simulink model "Underactuated_PFL_SMC"  (R2024b)
settings: Solver=FixedStepAuto  StartTime=0.0  StopTime=50  FixedStep=0.0001  RelTol=1e-3
settings Model: Creator=olive  LastModifiedBy=olivermcnaughton
settings DebuggingCC: UnderSpecifiedDimensionMsg=warning

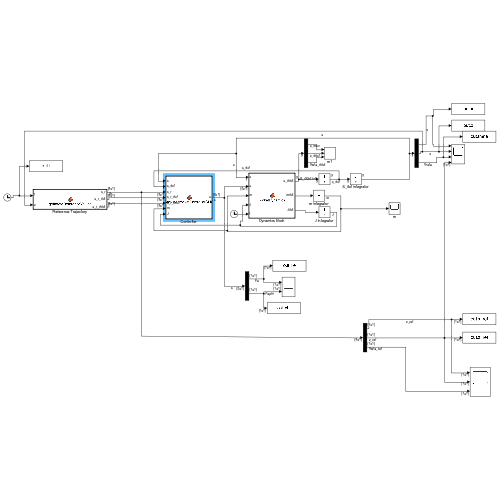
[thumbnail: Simulink's stored preview of the top-level diagram]
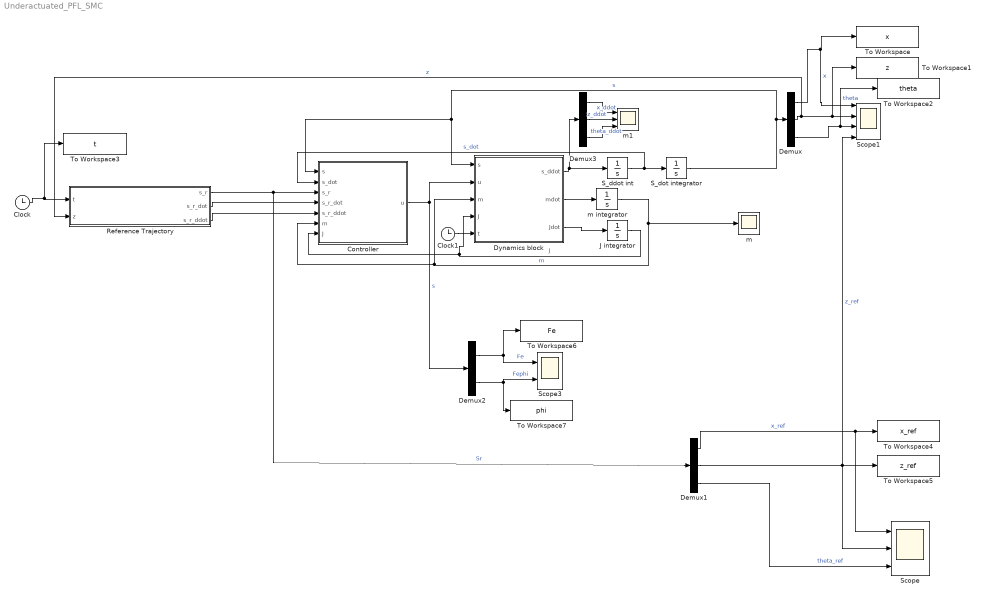
== system Underactuated_PFL_SMC ==
  Clock : Clock
  Clock1 : Clock
  Controller : MATLAB Function  TreatAsAtomicUnit=on
  Demux : Demux  Outputs=3
  Demux1 : Demux  Outputs=3
  Demux2 : Demux  Outputs=2
  Demux3 : Demux  Outputs=3
  Dynamics block : MATLAB Function  TreatAsAtomicUnit=on
  J integrator : Integrator  InitialCondition=5
  Reference Trajectory : MATLAB Function  TreatAsAtomicUnit=on
  S_ddot int : Integrator  InitialCondition=[0; 0; 0]
  S_dot integrator : Integrator  InitialCondition=[0;0;0]
  Scope : Scope  NumInputPorts=3
  Scope1 : Scope  NumInputPorts=4
  Scope3 : Scope  NumInputPorts=2
  To Workspace : ToWorkspace  VariableName=x  SaveFormat=Timeseries  SampleTime=-1
  To Workspace1 : ToWorkspace  VariableName=z  SaveFormat=Timeseries  SampleTime=-1
  To Workspace2 : ToWorkspace  VariableName=theta  SaveFormat=Timeseries  SampleTime=-1
  To Workspace3 : ToWorkspace  VariableName=t  SaveFormat=Timeseries  SampleTime=-1
  To Workspace4 : ToWorkspace  VariableName=x_ref  SaveFormat=Timeseries  SampleTime=-1
  To Workspace5 : ToWorkspace  VariableName=z_ref  SaveFormat=Timeseries  SampleTime=-1
  To Workspace6 : ToWorkspace  VariableName=Fe  SaveFormat=Timeseries  SampleTime=-1
  To Workspace7 : ToWorkspace  VariableName=phi  SaveFormat=Timeseries  SampleTime=-1
  m : Scope
  m integrator : Integrator  InitialCondition=25
  m1 : Scope  NumInputPorts=3
  wires:
  Dynamics block/1(s_ddot) -> Demux3/1, S_ddot int/1
  Dynamics block/2(mdot) -> m integrator/1
  Dynamics block/3(Jdot) -> J integrator/1
  S_ddot int/1 -> Controller/2(s_dot), S_dot integrator/1  "s_dot"
  S_dot integrator/1 -> Controller/1(s), Dynamics block/1(s), Demux/1  "s"
  J integrator/1 -> Dynamics block/4(J), Controller/7(J)  "J"
  m integrator/1 -> Dynamics block/3(m), Controller/6(m), m/1  "m"
  Demux/1 -> To Workspace/1, Scope1/1  "x"
  Demux/2 -> Reference Trajectory/2(z), To Workspace1/1, Scope1/2  "z"
  Demux/3 -> To Workspace2/1, Scope1/3  "theta"
  Demux2/2 -> To Workspace7/1, Scope3/2  "Fephi"
  Demux2/1 -> To Workspace6/1, Scope3/1  "Fe"
  Controller/1(u) -> Dynamics block/2(u), Demux2/1  "s"
  Clock/1 -> To Workspace3/1, Reference Trajectory/1(t)
  Reference Trajectory/1(s_r) -> Demux1/1, Controller/3(s_r)  "Sr"
  Demux1/2 -> To Workspace5/1, Scope1/4, Scope/2  "z_ref"
  Demux1/1 -> Scope/1, To Workspace4/1  "x_ref"
  Demux1/3 -> Scope/3  "theta_ref"
  Reference Trajectory/2(s_r_dot) -> Controller/4(s_r_dot)
  Demux3/1 -> m1/1  "x_ddot"
  Demux3/2 -> m1/2  "z_ddot"
  Demux3/3 -> m1/3  "theta_ddot"
  Reference Trajectory/3(s_r_ddot) -> Controller/5(s_r_ddot)
  Clock1/1 -> Dynamics block/5(t)

== matlab function Underactuated_PFL_SMC/Reference Trajectory ==
  data: s_r output; s_r_dot output; t input; z input; s_r_ddot output
function [s_r, s_r_dot, s_r_ddot] = generateReferenceValues(t,z)
% Generates constant reference position and velocity values for x, z, and theta
% Outputs:
%   sr: Reference position vector [x_ref; z_ref; theta_ref]
%   srdot: Reference velocity vector [x_dot_ref; z_dot_ref; theta_dot_ref]

%set position and time for each segment
%set to 1 for a hover, set 0 otherwise
hover = 1;
%set to 1 if tuning
if hover ==1
    x_ref = 2;
    z_ref = 2;
    theta_ref = 0;

    x_dot_ref = 0;
    z_dot_ref = 0;
    theta_dot_ref = 0;

    x_ddot_ref = 0;
    z_ddot_ref = 0;
    theta_ddot_ref = 0;
else
    %the rocket follows a trajectory of a half sine wave (middle part) then a
    %semi circle for the top of the boostback portion 
    %then a straight line downwards
    %End time of half sinewave
    T1 = 10;
    %End point of half sine wave
    x1 = 30;
    z1 = 40;
    
    %End time of semi circle 
    T2 = 20;
    %End point of semi circle
    x2 = 15; %gives you the position of the other side of the semi circle
    z2 = 40; %this should equal z1
    
    %Landing time of rocket
    T3 = 50;
    
    % Initialize reference values for safety
    x_ref = 0;
    z_ref = 0;
    theta_ref = 0;

    x_dot_ref = 0;
    z_dot_ref = 0;
    theta_dot_ref = 0;

    x_ddot_ref = 0;
    z_ddot_ref = 0;
    theta_ddot_ref = 0;

    %The first half sine wave
    if t<T1
        %reference positions
        x_ref = (-sin((pi/2) + pi*t/T1)+1)*x1/2;
        z_ref = z1*t/T1;
        theta_ref = atan(sin(pi*t/T1));
        
        %Reference Velocities
        x_dot_ref = (-pi/T1)*cos((pi/2) + pi*t/T1)*x1/2;
        z_dot_ref = z1/T1;
        theta_dot_ref = (pi/T1)*cos(pi*t/T1)/(sin(pi*t/T1)^2 + 1);

        %Reference Accelerations
        x_ddot_ref = ((pi/T1)^2)*sin((pi/2) + pi*t/T1)*x1/2;
        z_ddot_ref = 0;
        k = pi/T1;
        theta_ddot_ref = -k^2 * sin(k * t) * (3 - sin(k * t)^2) / (1 + sin(k * t)^2)^2;
    end
    %now doing the semi circle
    if t<T2 && t>=T1
        %calculate radius
        r = (x1-x2)/2; %radius 
        h = (x1+x2)/2; %x position for centre of circle
        dT = T2-T1; %Time between points
        dX = x1-x2;
        thetaMax = pi/4; %max angle at when halfway through the semi circle 
        teff = t -T1; %need to "zero" compared to the RHS of the semi circle
        %reference positions
        x_ref = h + r*cos(pi*teff/dT);
        z_ref = z1 + r*sin(pi*teff/dT);
        theta_ref = thetaMax*sin(2*pi*teff/dT + pi);
        %Reference Velocities
        x_dot_ref = (-pi/dT)*r*sin(pi*teff/dT);
        z_dot_ref = (pi/dT)*r*cos(pi*teff/dT);
        theta_dot_ref = thetaMax*(2*pi/dT)*cos(2*pi*teff/dT + pi);

        %Reference Accelerations
        x_ddot_ref = -(pi^2/dT^2)*r*cos(pi*teff/dT);
        z_ddot_ref = -(pi^2/dT^2)*r*sin(pi*teff/dT);
        theta_ddot_ref = -4*(pi^2/dT^2)*thetaMax*sin(pi*teff/dT + pi);
    end
    %now it is landing
    if t>=T2 
        % Position
        x_ref = x2; % Assuming no horizontal movement during landing
        z_ref = z2-4*(t-T2);
        theta_ref = 0; % No rotation during landing
        
        % Velocity
        x_dot_ref = 0;
        if z<10
            z_dot_ref = 0;
            z_ref = 5;
        else 
            z_dot_ref = -4;
        end
        
        theta_dot_ref = 0;
        
        % Acceleration
        x_ddot_ref = 0;
        z_ddot_ref = 0;
        theta_ddot_ref = 0;
    end
    if t>T3
        x_ref = x2;
        z_ref = 5;
        theta_ref = 0; % No rotation during landing
    end
    
end
% Output reference values
s_r = [x_ref; z_ref; theta_ref];
s_r_dot = [x_dot_ref; z_dot_ref; theta_dot_ref];
s_r_ddot = [x_ddot_ref; z_ddot_ref; theta_ddot_ref];
end

== matlab function Underactuated_PFL_SMC/Dynamics block ==
  data: s input size=3; u input; m input; J input; s_ddot output size=3; mdot output size=1; Jdot output size=1; t input
function [s_ddot,mdot,Jdot] = rocketDynamics(s,u,m,J,t)

%initialise states
L1 = 1;
alpha1 = 0.009;
alpha2 = 0.005;
beta = 0.03;
g = 9.81;

%extract states
Fe = u(1);
phi = u(2);
theta = s(3);

%find mdot and Jdot
mdot = -alpha1*(beta*Fe);
Jdot = -alpha2*(beta*Fe);

% Disturbances 
Fx_dist = 20*sin(0.5*t);    %N     
Fz_dist = 20*sin(0.5*t);    %N
M_dist  = 20*sin(0.5*t);    %(Nm)

% Maybe the actual mass is 20% heavier than the "m" we pass to the controller
m_actual = 1 * m; 

%acclerations 
x_ddot     = (Fe*sin(theta + phi) + Fx_dist) / m_actual;
z_ddot     = -g + (Fe*cos(theta + phi) + Fz_dist) / m_actual;
theta_ddot = (Fe*sin(phi)*L1 + M_dist) / J;

s_ddot = [x_ddot;z_ddot;theta_ddot];

end

== matlab function Underactuated_PFL_SMC/Controller ==
  data: s input; s_dot input; s_r input; s_r_dot input; s_r_ddot input; m input; J input; u output
function u = BacksteprocketControllerSMC(s, s_dot, s_r, s_r_dot, s_r_ddot, m, J)
% rocketController - Backstepping-based + Sliding Mode Control for rocket dynamics

% Define bounds
FE_min = 0;   % Lower bound for FE
FE_max = 500; % Upper bound for FE
phi_min = -pi/6;  % Lower bound for phi
phi_max = pi/6;   % Upper bound for phi

% Constants
g = 9.81; % Gravity

% Extract current states
x = s(1);
z = s(2);
theta = s(3);
x_dot = s_dot(1);
z_dot = s_dot(2);
theta_dot = s_dot(3);

% Extract reference states
x_ref = s_r(1);
z_ref = s_r(2);
theta_ref = s_r(3);
x_dot_ref = s_r_dot(1);
z_dot_ref = s_r_dot(2);
theta_dot_ref = s_r_dot(3);
x_ddot_ref = s_r_ddot(1);
z_ddot_ref = s_r_ddot(2);
theta_ddot_ref = s_r_ddot(3);

% Control gains (Backstepping)
%proportional | Derivative
kpx = 2;        kdx = 5;
kpz = 2;        kdz = 5;
kpt = 1;        kdt = 1;

% Sliding Mode Gains
lambda_x = 0.1;  % Tuning parameter for x sliding surface
lambda_z = 0.1;  % Tuning parameter for z sliding surface
lambda_t = 0.1;  % Tuning parameter for theta sliding surface

eta_x = 10;    % SMC gain for x
eta_z = 0.1;    % SMC gain for z
eta_t = 0.1;     % SMC gain for theta

psi_x = 1;
psi_z = 1;
psi_t = 1;

% Define Sliding Surfaces
ex = x - x_ref;
ez = z - z_ref;
et = theta - theta_ref;
edotx = x_dot - x_dot_ref;
edotz = z_dot - z_dot_ref;
edot_t = theta_dot - theta_dot_ref;

sx = edotx + lambda_x * ex;  % Sliding surface for x
sz = edotz + lambda_z * ez;  % Sliding surface for z
st = edot_t + lambda_t * et; % Sliding surface for theta

% Smooth Sliding Mode Control (Using Tanh Function)
SMC_x = -eta_x * tanh(sx / psi_x);
SMC_z = -eta_z * tanh(sz / psi_z);
SMC_t = -eta_t * tanh(st / psi_t);

%PD controller 
ax_PD = - kpx * ex - kdx * edotx;
az_PD = - kpz * ez - kdz * edotz;
t_PD = - kpt * et - kdt * edot_t;

% Desired acceleration (Modified with SMC)
ax = x_ddot_ref + ax_PD + SMC_x;
az = z_ddot_ref + az_PD + SMC_z;

% Avoid division by zero
denominator = az + g;
if abs(denominator) < 1e-6
    denominator = sign(denominator) * 1e-6;
end

% Compute control inputs
phi_ff = atan2(ax, denominator) - theta; %Feedforward phi (even though it contains feedback in the x/y accelerations it does not count as feedback)
Fe = m * sqrt(ax^2 + (az + g)^2); 
phi = phi_ff + t_PD + SMC_t;  % Outer Loop Control, remember u = ueq + usmc 

% Bound within physical limits
Fe = max(FE_min, min(Fe, FE_max));
phi = max(phi_min, min(phi, phi_max));

% Output control vector
u = [Fe; phi];

end
